simulink model "admire_sim_NDI"  (Simulink 9.1)
settings: Solver=ode4  StartTime=0.0  StopTime=500  FixedStep=dt  RelTol=1e-3  AbsTol=1e-6
InitFcn:
  | INIT_NDI
StartFcn:
  | tic
StopFcn:
  | toctime=toc;
  | fprintf('Actual Time = %g\nSim Time = %g\n',toctime,tout(end))
  | % Make plots
  | %admire_sim_plot
  | figure
  | plot3(yout(:,11),yout(:,10),-yout(:,12),'*-');grid
  | xlabel('East (m)');ylabel('North (m)');zlabel('Alt (m)')
  | view([0 0 1])
  | hold on
  | plot3(Ywpt,Xwpt,0*Xwpt,'r^-','MarkerSize',10)
  | axis equal
  | hold off
values from neighbouring files (symbols this model uses):
  a1 = (180*d2r)/(80^3)    (= 6.13592315154e-06)    [INIT_NDI.m]
  a2 = (24*d2r)/(80^3)    (= 8.18123086872e-07)    [INIT_NDI.m]
  Altcmd_t = [ 0    1   100 200  300  425  450  550  600  700  800  880  980]    [INIT_NDI.m]
  Altcmd_v = [20  20   20   1500 1500 1500 1500 3000 3000 4000 4000 6000 6000]    [INIT_NDI.m]
  bref = 10    [INIT_NDI.m]
  C1 = ((Iy-Iz)*Iz-Ixz^2)/GG    (= -0.958151081688)    [INIT_NDI.m]
  C2 = (Ix-Iy+Iz)*Ixz/GG    (= 0.0484690861804)    [INIT_NDI.m]
  C3 = Iz/GG    (= 4.77597824802e-05)    [INIT_NDI.m]
  C4 = Ixz/GG    (= 1.18217283367e-06)    [INIT_NDI.m]
  C5 = (Iz-Ix)/Iy    (= 0.987654320988)    [INIT_NDI.m]
  C6 = Ixz/Iy    (= 0.0308641975309)    [INIT_NDI.m]
  C7 = 1/Iy    (= 1.23456790123e-05)    [INIT_NDI.m]
  C8 = (Ix*(Ix-Iy)+Ixz^2)/GG    (= -0.592859676085)    [INIT_NDI.m]
  C9 = Ix/GG    (= 9.93025180281e-06)    [INIT_NDI.m]
  CAmethod = 6    [INIT_NDI.m]
  Canard_max = [25 25 25 15 15 15 15 15]*d2r    [INIT_NDI.m]
  Canard_min = [-55 -55 -25 -15 -15 -15 -15 -15]*d2r    [INIT_NDI.m]
  CB = CCV*Bbare    [INIT_NDI.m]
  CC = [C3 0 C4;0 C7 0;C4 0 C9]    [INIT_NDI.m]
  CCV = [CCV zeros(3,22)]    [INIT_NDI.m]
  cref = 5.2    [INIT_NDI.m]
  d2r = pi/180    (= 0.0174532925199)    [INIT_NDI.m]
  dt = 0.01    [INIT_NDI.m]
  DTY_max = 0.002    [INIT_NDI.m]
  DTY_min = -0.002    [INIT_NDI.m]
  DTZ_max = 0.002    [INIT_NDI.m]
  DTZ_min = -0.002    [INIT_NDI.m]
  du = [eye(7,7)*d2r eye(7,7)*(-d2r);zeros(20,14)]    [INIT_NDI.m]
  Elevon_max = [30 30 25 25 25 25 25 25]*d2r    [INIT_NDI.m]
  Elevon_min = [-30 -30 -30 -30 -30 -30 -30 -30]*d2r    [INIT_NDI.m]
  G = [ 0 1 0 ... (first row only)    [INIT_NDI.m]
  kcb = 2.5    [INIT_NDI.m]
  kfb = -0.4    [INIT_NDI.m]
  kib = 0.2    [INIT_NDI.m]
  kpb = 0.8    [INIT_NDI.m]
  LEF_max = [30 30 30 20 20 15 10 10]*d2r    [INIT_NDI.m]
  LEF_min = [-10 -10 -10 -10 -10 -10 -10 -10]*d2r    [INIT_NDI.m]
  LG_max = 1    [INIT_NDI.m]
  LG_min = 0    [INIT_NDI.m]
  LPmethod = 5    [INIT_NDI.m]    (also in LPwrap.m = 0)
  M_vec = [0 0.5 0.8 0.9 0.95 1.4 1.5 2.5]    [INIT_NDI.m]
  mass = 9100    [INIT_NDI.m]
  NumU = 16    [INIT_NDI.m]
  nwpt = 5    [INIT_NDI.m]
  PD_max = 10    [INIT_NDI.m]
  PD_min = -10    [INIT_NDI.m]
  PHIcmd_t = [0 1 1+dt 30 30+dt 60 60+dt 90 90+dt 120 120+dt 150 150+dt 180 180+dt 210 210+dt 240 240+dt 270 270+dt 300 300+dt 330 330+dt]    [INIT_NDI.m]
  PHIcmd_v = [0 0 15   15 -15   -15 0    0   30   30  -30    -30 0      0   45     45   0     0    -45   -45   0     0   -60   -60 0]    [INIT_NDI.m]
  Pmode = 3    [INIT_NDI.m]
  r2d = 180/pi    (= 57.2957795131)    [INIT_NDI.m]
  Rmode = 3    [INIT_NDI.m]
  Rudder_max = [30 30 25 20 15 15 15 10]*d2r    [INIT_NDI.m]
  Rudder_min = [-30 -30 -25 -20 -15 -15 -15 -10]*d2r    [INIT_NDI.m]
  Sref = 45    [INIT_NDI.m]
  TSS_max = 1    [INIT_NDI.m]
  TSS_min = 0    [INIT_NDI.m]
  UD_max = 10    [INIT_NDI.m]
  UD_min = -10    [INIT_NDI.m]
  Upref = [0 0 0 0 0 0 0 0 0 0 0 0 0 0 0 0]'    [INIT_NDI.m]
  Upref_split = [[0 0 30 -30 -30 30 0]*d2r*.4 0 0 0 0 0 0 0 0 0]'    [INIT_NDI.m]
  Urlim = [50*d2r ... (first row only)    [INIT_NDI.m]
  UseRL = 0    [INIT_NDI.m]
  Vcmd_t = [  0    1   100  200  300  425  450  550  600  700  800  880  980]    [INIT_NDI.m]
  Vcmd_v = Mcmd_v.*a    [INIT_NDI.m]
  VD_max = 10    [INIT_NDI.m]
  VD_min = -10    [INIT_NDI.m]
  WD_max = 10    [INIT_NDI.m]
  WD_min = -10    [INIT_NDI.m]
  Wp = W'*W    [INIT_NDI.m]
  Wpts = [0 1 2 3 4]    [INIT_NDI.m]
  x0 = [ max(eyp,zeros(n,1));max(-eyp,zeros(n,1));zeros(2*m,1)]    [LPwrap.m]
  Xwpt = [0 4000 4000 0 0]*8    [INIT_NDI.m]
  Ywpt = [0 0 4000 4000 0]*8    [INIT_NDI.m]
undefined symbols (not defined in the file or in its folder): Abare, Bbare, CGIwrap, dalpha_err, dalt_err, DAwrap, dbeta_err, ddc_bw, ddc_rate, ddei_bw, ddei_rate, ddey_bw, ddey_rate, ddle_bw, ddle_rate, ddr_bw, ddr_rate, DiscIntNeverNeededParam, dVt_err, LPwrap, rlimit_c, rlimit_ie, rlimit_le, rlimit_oe, rlimit_r, u0fcs, u0new, VJAwrap, x0bare, y0bare
libraries: simulink_extras x19, simulink x12
(part 4 of 4)

== system admire_sim_NDI/NDI_CLAW/DynamicInversionControl/AERO_OBM/NonLinearOBM/Get_B_Aero/OneColPerFrame/u4 ==
  In1 : Inport
  Action Port : ActionPort  ActionType=case
  ADMIRE_aerotesthigh : S-Function  FunctionName=admire_aerotesthigh  SFunctionDeploymentMode=off  EnableBusSupport=off
  ADMIRE_aerotesthigh1 : S-Function  FunctionName=admire_aerotesthigh  SFunctionDeploymentMode=off  EnableBusSupport=off
  Constant1 : Constant  Value=zeros(25,1)
  Gain : Gain  Gain=0.5*r2d
  Selector : Selector  NumberOfDimensions=2  InputPortWidth=3  IndexOptions=Index vector (dialog),Index vector (dialog)  Indices=[1:27],4  OutputSizes=1,1
  Selector1 : Selector  NumberOfDimensions=2  InputPortWidth=3  IndexOptions=Index vector (dialog),Index vector (dialog)  Indices=[1:27],11  OutputSizes=1,1
  Selector2 : Selector  InputPortWidth=9  IndexOptions=Index vector (dialog)  Indices=[4:6]  OutputSizes=1
  Selector3 : Selector  InputPortWidth=9  IndexOptions=Index vector (dialog)  Indices=[4:6]  OutputSizes=1
  Sum1 : Sum  Inputs=|+-
  Out1 : Outport
  wires:
  Constant1/1 -> ADMIRE_aerotesthigh/2, ADMIRE_aerotesthigh1/2
  In1/1 -> Selector1/1, Selector/1
  Selector/1 -> ADMIRE_aerotesthigh/1
  Selector1/1 -> ADMIRE_aerotesthigh1/1
  ADMIRE_aerotesthigh/1 -> Selector2/1
  ADMIRE_aerotesthigh1/1 -> Selector3/1
  Sum1/1 -> Gain/1
  Selector2/1 -> Sum1/1
  Selector3/1 -> Sum1/2
  Gain/1 -> Out1/1

== system admire_sim_NDI/NDI_CLAW/DynamicInversionControl/AERO_OBM/NonLinearOBM/Get_B_Aero/OneColPerFrame/u5 ==
  In1 : Inport
  Action Port : ActionPort  ActionType=case
  ADMIRE_aerotesthigh : S-Function  FunctionName=admire_aerotesthigh  SFunctionDeploymentMode=off  EnableBusSupport=off
  ADMIRE_aerotesthigh1 : S-Function  FunctionName=admire_aerotesthigh  SFunctionDeploymentMode=off  EnableBusSupport=off
  Constant1 : Constant  Value=zeros(25,1)
  Gain : Gain  Gain=0.5*r2d
  Selector : Selector  NumberOfDimensions=2  InputPortWidth=3  IndexOptions=Index vector (dialog),Index vector (dialog)  Indices=[1:27],5  OutputSizes=1,1
  Selector1 : Selector  NumberOfDimensions=2  InputPortWidth=3  IndexOptions=Index vector (dialog),Index vector (dialog)  Indices=[1:27],12  OutputSizes=1,1
  Selector2 : Selector  InputPortWidth=9  IndexOptions=Index vector (dialog)  Indices=[4:6]  OutputSizes=1
  Selector3 : Selector  InputPortWidth=9  IndexOptions=Index vector (dialog)  Indices=[4:6]  OutputSizes=1
  Sum1 : Sum  Inputs=|+-
  Out1 : Outport
  wires:
  Gain/1 -> Out1/1
  Selector3/1 -> Sum1/2
  Selector2/1 -> Sum1/1
  Sum1/1 -> Gain/1
  ADMIRE_aerotesthigh1/1 -> Selector3/1
  ADMIRE_aerotesthigh/1 -> Selector2/1
  Selector1/1 -> ADMIRE_aerotesthigh1/1
  Selector/1 -> ADMIRE_aerotesthigh/1
  In1/1 -> Selector/1, Selector1/1
  Constant1/1 -> ADMIRE_aerotesthigh/2, ADMIRE_aerotesthigh1/2

== system admire_sim_NDI/NDI_CLAW/DynamicInversionControl/AERO_OBM/NonLinearOBM/Get_B_Aero/OneColPerFrame/u6 ==
  In1 : Inport
  Action Port : ActionPort  ActionType=case
  ADMIRE_aerotesthigh : S-Function  FunctionName=admire_aerotesthigh  SFunctionDeploymentMode=off  EnableBusSupport=off
  ADMIRE_aerotesthigh1 : S-Function  FunctionName=admire_aerotesthigh  SFunctionDeploymentMode=off  EnableBusSupport=off
  Constant1 : Constant  Value=zeros(25,1)
  Gain : Gain  Gain=0.5*r2d
  Selector : Selector  NumberOfDimensions=2  InputPortWidth=3  IndexOptions=Index vector (dialog),Index vector (dialog)  Indices=[1:27],6  OutputSizes=1,1
  Selector1 : Selector  NumberOfDimensions=2  InputPortWidth=3  IndexOptions=Index vector (dialog),Index vector (dialog)  Indices=[1:27],13  OutputSizes=1,1
  Selector2 : Selector  InputPortWidth=9  IndexOptions=Index vector (dialog)  Indices=[4:6]  OutputSizes=1
  Selector3 : Selector  InputPortWidth=9  IndexOptions=Index vector (dialog)  Indices=[4:6]  OutputSizes=1
  Sum1 : Sum  Inputs=|+-
  Out1 : Outport
  wires:
  Constant1/1 -> ADMIRE_aerotesthigh/2, ADMIRE_aerotesthigh1/2
  In1/1 -> Selector1/1, Selector/1
  Selector/1 -> ADMIRE_aerotesthigh/1
  Selector1/1 -> ADMIRE_aerotesthigh1/1
  ADMIRE_aerotesthigh/1 -> Selector2/1
  ADMIRE_aerotesthigh1/1 -> Selector3/1
  Sum1/1 -> Gain/1
  Selector2/1 -> Sum1/1
  Selector3/1 -> Sum1/2
  Gain/1 -> Out1/1

== system admire_sim_NDI/NDI_CLAW/DynamicInversionControl/AERO_OBM/NonLinearOBM/Get_B_Aero/OneColPerFrame/u7 ==
  In1 : Inport
  Action Port : ActionPort  ActionType=case
  ADMIRE_aerotesthigh : S-Function  FunctionName=admire_aerotesthigh  SFunctionDeploymentMode=off  EnableBusSupport=off
  ADMIRE_aerotesthigh1 : S-Function  FunctionName=admire_aerotesthigh  SFunctionDeploymentMode=off  EnableBusSupport=off
  Constant1 : Constant  Value=zeros(25,1)
  Gain : Gain  Gain=0.5*r2d
  Selector : Selector  NumberOfDimensions=2  InputPortWidth=3  IndexOptions=Index vector (dialog),Index vector (dialog)  Indices=[1:27],7  OutputSizes=1,1
  Selector1 : Selector  NumberOfDimensions=2  InputPortWidth=3  IndexOptions=Index vector (dialog),Index vector (dialog)  Indices=[1:27],14  OutputSizes=1,1
  Selector2 : Selector  InputPortWidth=9  IndexOptions=Index vector (dialog)  Indices=[4:6]  OutputSizes=1
  Selector3 : Selector  InputPortWidth=9  IndexOptions=Index vector (dialog)  Indices=[4:6]  OutputSizes=1
  Sum1 : Sum  Inputs=|+-
  Out1 : Outport
  wires:
  Gain/1 -> Out1/1
  Selector3/1 -> Sum1/2
  Selector2/1 -> Sum1/1
  Sum1/1 -> Gain/1
  ADMIRE_aerotesthigh1/1 -> Selector3/1
  ADMIRE_aerotesthigh/1 -> Selector2/1
  Selector1/1 -> ADMIRE_aerotesthigh1/1
  Selector/1 -> ADMIRE_aerotesthigh/1
  In1/1 -> Selector/1, Selector1/1
  Constant1/1 -> ADMIRE_aerotesthigh/2, ADMIRE_aerotesthigh1/2

== system admire_sim_NDI/NDI_CLAW/DynamicInversionControl/ControlAllocation/GetU/WeightedPseudo Scaled_2/Blocks/CheckSaturation ==
  In1 : Inport
  Umin : Inport  Port=2
  Umax : Inport  Port=3
  Relational Operator : RelationalOperator  Operator=<  OutDataTypeStr=boolean  RndMeth=Nearest
  Relational Operator1 : RelationalOperator  Operator=>  OutDataTypeStr=boolean  RndMeth=Nearest
  Sum : Sum  Inputs=|++
  Sum of Elements : Sum  Inputs=+
  Sum of Elements1 : Sum  Inputs=+
  Out1 : Outport
  wires:
  Sum/1 -> Out1/1
  In1/1 -> Relational Operator/1, Relational Operator1/1
  Sum of Elements1/1 -> Sum/2
  Sum of Elements/1 -> Sum/1
  Relational Operator/1 -> Sum of Elements1/1
  Relational Operator1/1 -> Sum of Elements/1
  Umax/1 -> Relational Operator1/2
  Umin/1 -> Relational Operator/2

== system admire_sim_NDI/NDI_CLAW/DynamicInversionControl/ControlAllocation/GetU/WeightedPseudo Scaled_2/Blocks/GetP ==
  CB : Inport
  WpT : Inport  Port=2
  CBT : Inport  Port=3
  Product : Product  Inputs=/*  Multiplication=Matrix(*)  RndMeth=Zero
  Product1 : Product  Inputs=**  Multiplication=Matrix(*)  RndMeth=Zero
  Product2 : Product  Inputs=*/  Multiplication=Matrix(*)  RndMeth=Zero
  P : Outport
  wires:
  CBT/1 -> Product/2
  Product2/1 -> P/1  "P"
  WpT/1 -> Product/1
  CB/1 -> Product1/1
  Product1/1 -> Product2/2
  Product/1 -> Product2/1, Product1/2

== system admire_sim_NDI/NDI_CLAW/DynamicInversionControl/ControlAllocation/GetU/WeightedPseudo Scaled_2/Blocks/None_Saturated ==
  In1 : Inport
  Action Port : ActionPort  ActionType=then
  Out1 : Outport
  wires:
  In1/1 -> Out1/1

== system admire_sim_NDI/NDI_CLAW/DynamicInversionControl/ControlAllocation/GetU/WeightedPseudo Scaled_2/Blocks/Some_Saturated ==
  umax : Inport
  umin : Inport  Port=2
  u : Inport  Port=3
  Action Port : ActionPort  ActionType=else
  For Iterator Subsystem : Subsystem  TreatAsAtomicUnit=on
  Product : Product  RndMeth=Zero
  Out1 : Outport
  wires:
  Product/1 -> Out1/1
  For Iterator Subsystem/1(Out1) -> Product/2
  umin/1 -> For Iterator Subsystem/3(umin)
  umax/1 -> For Iterator Subsystem/2(umax)
  u/1 -> Product/1, For Iterator Subsystem/1(u)

== system admire_sim_NDI/NDI_CLAW/DynamicInversionControl/ControlAllocation/PostProcess/DriveToPreferred/LimitScale/Calculate the gain factor to the lower limit  ==
  oou : Inport
  MaxValues : Inport  Port=2
  PrePro : Inport  Port=3
  Bus Selector2 : BusSelector  OutputSignals=INDX
  Compare To Constant : simulink/Logic and Bit Operations/Compare To Constant  relop=<=  const=0.5  OutDataTypeStr=uint8
  Data Type Conversion : DataTypeConversion  OutDataTypeStr=double
  Product : Product  Inputs=*/  RndMeth=Zero
  Product2 : Product
  Sum : Sum  Inputs=|++
  Out1 : Outport
  wires:
  Compare To Constant/1 -> Data Type Conversion/1
  Data Type Conversion/1 -> Sum/1
  Bus Selector2/1 -> Product2/1, Compare To Constant/1  "<INDX>"
  Product2/1 -> Sum/2
  PrePro/1 -> Bus Selector2/1
  MaxValues/1 -> Product/1
  Sum/1 -> Out1/1
  oou/1 -> Product/2
  Product/1 -> Product2/2  "gain,  K"

== system admire_sim_NDI/NDI_CLAW/DynamicInversionControl/ControlAllocation/PostProcess/DriveToPreferred/LimitScale/Calculate the gain factor to the upper limit  ==
  PrePro : Inport
  MinValues : Inport  Port=2
  oou : Inport  Port=3
  Bus Selector2 : BusSelector  OutputSignals=INDX
  Compare To Constant : simulink/Logic and Bit Operations/Compare To Constant  relop=<=  const=0.5  OutDataTypeStr=uint8
  Data Type Conversion : DataTypeConversion  OutDataTypeStr=double
  Product : Product  Inputs=*/  RndMeth=Zero
  Product2 : Product
  Sum : Sum  Inputs=|++
  Out1 : Outport
  wires:
  Product/1 -> Product2/2
  oou/1 -> Product/2
  Sum/1 -> Out1/1
  MinValues/1 -> Product/1
  PrePro/1 -> Bus Selector2/1
  Product2/1 -> Sum/2
  Bus Selector2/1 -> Product2/1, Compare To Constant/1  "<INDX>"
  Data Type Conversion/1 -> Sum/1
  Compare To Constant/1 -> Data Type Conversion/1

== system admire_sim_NDI/NDI_CLAW/DynamicInversionControl/ControlAllocation/PostProcess/DriveToPreferred/LimitScale/DivideByZeroProtection ==
  In1 : Inport
  Abs : Abs
  Compare To Constant : simulink/Logic and Bit Operations/Compare To Constant  relop=<=  const=1e-5  OutDataTypeStr=uint8
  Compare To Zero : simulink/Logic and Bit Operations/Compare To Zero  relop=>=  OutDataTypeStr=uint8
  Constant : Constant
  Data Type Conversion : DataTypeConversion  OutDataTypeStr=double
  Data Type Conversion1 : DataTypeConversion  OutDataTypeStr=double
  Gain1 : Gain  Gain=1e-5
  Gain2 : Gain  Gain=2
  Product1 : Product  RndMeth=Zero
  Sum : Sum  Inputs=|++
  Sum1 : Sum  Inputs=|+-
  Out1 : Outport
  wires:
  Abs/1 -> Compare To Constant/1
  Data Type Conversion/1 -> Gain1/1
  Gain1/1 -> Product1/1
  Sum1/1 -> Data Type Conversion1/1
  Compare To Zero/1 -> Gain2/1
  Gain2/1 -> Sum1/1
  Constant/1 -> Sum1/2
  Data Type Conversion1/1 -> Product1/2
  Compare To Constant/1 -> Data Type Conversion/1
  In1/1 -> Sum/1, Compare To Zero/1, Abs/1
  Product1/1 -> Sum/2
  Sum/1 -> Out1/1

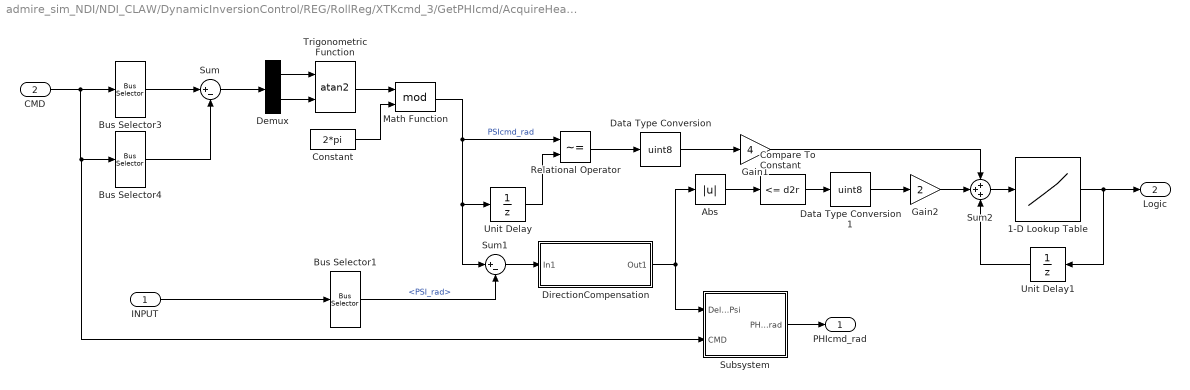
== system admire_sim_NDI/NDI_CLAW/DynamicInversionControl/REG/RollReg/XTKcmd_3/GetPHIcmd/AcquireHeading ==
  INPUT : Inport
  CMD : Inport  Port=2
  1-D Lookup Table : Lookup_n-D  NumberOfTableDimensions=1  BreakpointsForDimension1=[0 1 2 3 4 5 6 7]  Table=[0 1 0 0 1 1 1 1]  InterpMethod=Flat  OutDataTypeStr=uint8  RndMeth=Simplest  InputSameDT=on
  Abs : Abs
  Bus Selector1 : BusSelector  OutputSignals=PSI_rad
  Bus Selector3 : BusSelector  OutputSignals=Ycmd,Xcmd  OutputAsBus=on
  Bus Selector4 : BusSelector  OutputSignals=Ycmdm1,Xcmdm1  OutputAsBus=on
  Compare To Constant : simulink/Logic and Bit Operations/Compare To Constant  relop=<=  const=d2r  OutDataTypeStr=uint8
  Constant : Constant  Value=2*pi
  Data Type Conversion : DataTypeConversion  OutDataTypeStr=uint8
  Data Type Conversion1 : DataTypeConversion  OutDataTypeStr=uint8
  Demux : Demux  Outputs=2
  DirectionCompensation : Subsystem
  Gain1 : Gain  Gain=4  OutDataTypeStr=uint8
  Gain2 : Gain  Gain=2  OutDataTypeStr=uint8
  Math Function : Math  Operator=mod  SaturateOnIntegerOverflow=on
  Relational Operator : RelationalOperator  Operator=~=  OutDataTypeStr=boolean  RndMeth=Nearest
  Subsystem : Subsystem
  Sum : Sum  Inputs=|+-
  Sum1 : Sum  Inputs=|+-
  Sum2 : Sum  Inputs=+++
  Trigonometric Function : Trigonometry  Operator=atan2
  Unit Delay : UnitDelay  SampleTime=-1
  Unit Delay1 : UnitDelay  SampleTime=-1
  PHIcmd_rad : Outport
  Logic : Outport  Port=2
  wires:
  CMD/1 -> Subsystem/2(CMD), Bus Selector4/1, Bus Selector3/1
  INPUT/1 -> Bus Selector1/1
  Bus Selector3/1 -> Sum/1
  Bus Selector4/1 -> Sum/2
  Sum/1 -> Demux/1
  Demux/1 -> Trigonometric Function/1
  Demux/2 -> Trigonometric Function/2
  Trigonometric Function/1 -> Math Function/1
  Bus Selector1/1 -> Sum1/2  "<PSI_rad>"
  Math Function/1 -> Unit Delay/1, Sum1/1, Relational Operator/1  "PSIcmd_rad"
  Sum1/1 -> DirectionCompensation/1(In1)
  DirectionCompensation/1(Out1) -> Subsystem/1(DeltaPsi), Abs/1
  Constant/1 -> Math Function/2
  Unit Delay/1 -> Relational Operator/2
  Relational Operator/1 -> Data Type Conversion/1
  Abs/1 -> Compare To Constant/1
  Compare To Constant/1 -> Data Type Conversion1/1
  Sum2/1 -> 1-D Lookup Table/1
  Data Type Conversion/1 -> Gain1/1
  Gain1/1 -> Sum2/1
  Gain2/1 -> Sum2/2
  Data Type Conversion1/1 -> Gain2/1
  Unit Delay1/1 -> Sum2/3
  1-D Lookup Table/1 -> Logic/1, Unit Delay1/1
  Subsystem/1(PHIcmd_rad) -> PHIcmd_rad/1

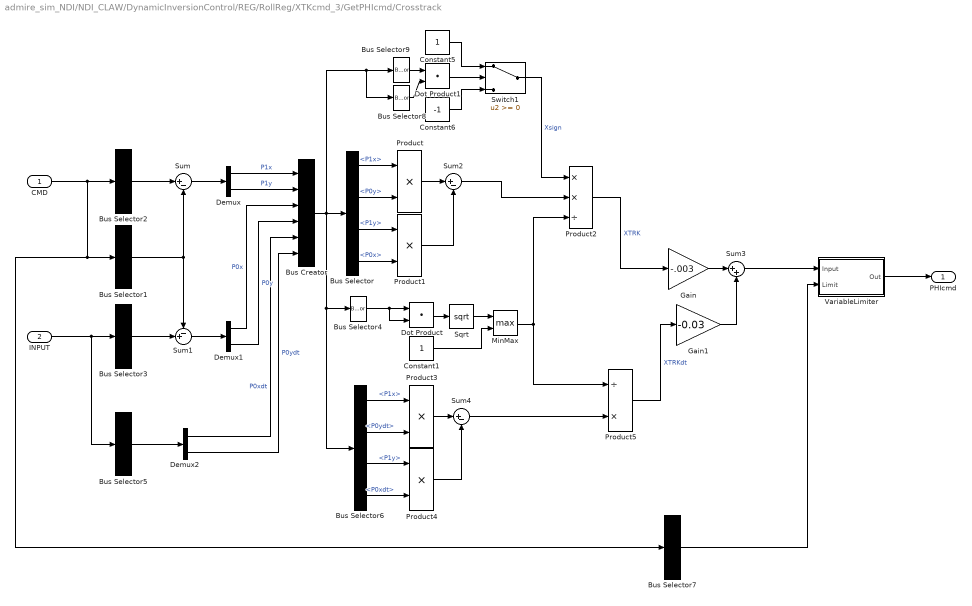
== system admire_sim_NDI/NDI_CLAW/DynamicInversionControl/REG/RollReg/XTKcmd_3/GetPHIcmd/Crosstrack ==
  CMD : Inport
  INPUT : Inport  Port=2
  Bus Creator : BusCreator  Inputs=6
  Bus Selector : BusSelector  OutputSignals=P1x,P0y,P1y,P0x
  Bus Selector1 : BusSelector  OutputSignals=Xcmdm1,Ycmdm1  OutputAsBus=on
  Bus Selector2 : BusSelector  OutputSignals=Xcmd,Ycmd  OutputAsBus=on
  Bus Selector3 : BusSelector  OutputSignals=X_m,Y_m  OutputAsBus=on
  Bus Selector4 : BusSelector  OutputSignals=P1x,P1y  OutputAsBus=on
  Bus Selector5 : BusSelector  OutputSignals=XV_mps,YV_mps  OutputAsBus=on
  Bus Selector6 : BusSelector  OutputSignals=P1x,P0ydt,P1y,P0xdt
  Bus Selector7 : BusSelector  OutputSignals=PHImax_rad  OutputAsBus=on
  Bus Selector8 : BusSelector  OutputSignals=P0xdt,P0ydt  OutputAsBus=on
  Bus Selector9 : BusSelector  OutputSignals=P1x,P1y  OutputAsBus=on
  Constant1 : Constant
  Constant5 : Constant
  Constant6 : Constant  Value=-1
  Demux : Demux  Outputs=2
  Demux1 : Demux  Outputs=2
  Demux2 : Demux  Outputs=2
  Dot Product : DotProduct  InputSameDT=on  OutDataTypeStr=Inherit: Inherit via internal rule
  Dot Product1 : DotProduct  InputSameDT=on  OutDataTypeStr=Inherit: Inherit via internal rule
  Gain : Gain  Gain=-.003
  Gain1 : Gain  Gain=-0.03
  MinMax : MinMax  Function=max  Inputs=2
  Product{,1,3..4} (4 alike) : Product  RndMeth=Zero
  Product2 : Product  Inputs=**/  RndMeth=Zero
  Product5 : Product  Inputs=/*  RndMeth=Zero
  Sqrt : Sqrt  SaturateOnIntegerOverflow=on
  Sum : Sum  Inputs=|+-
  Sum1 : Sum  Inputs=-+|
  Sum2 : Sum  Inputs=|+-
  Sum3 : Sum  Inputs=|++
  Sum4 : Sum  Inputs=|+-
  Switch1 : Switch
  VariableLimiter : Subsystem
  PHIcmd : Outport
  wires:
  CMD/1 -> Bus Selector2/1, Bus Selector1/1, Bus Selector7/1
  Bus Selector2/1 -> Sum/1
  Bus Selector1/1 -> Sum/2, Sum1/1
  INPUT/1 -> Bus Selector3/1, Bus Selector5/1
  Bus Selector3/1 -> Sum1/2
  Sum/1 -> Demux/1
  Sum1/1 -> Demux1/1
  Demux/1 -> Bus Creator/1  "P1x"
  Demux/2 -> Bus Creator/2  "P1y"
  Demux1/1 -> Bus Creator/3  "P0x"
  Demux1/2 -> Bus Creator/4  "P0y"
  Bus Creator/1 -> Bus Selector/1, Bus Selector4/1, Bus Selector6/1, Bus Selector9/1, Bus Selector8/1
  Bus Selector/1 -> Product/1  "<P1x>"
  Bus Selector/2 -> Product/2  "<P0y>"
  Bus Selector/3 -> Product1/1  "<P1y>"
  Bus Selector/4 -> Product1/2  "<P0x>"
  Product/1 -> Sum2/1
  Product1/1 -> Sum2/2
  Bus Selector4/1 -> Dot Product/1, Dot Product/2
  Dot Product/1 -> Sqrt/1
  Sqrt/1 -> MinMax/1
  Constant1/1 -> MinMax/2
  MinMax/1 -> Product5/1, Product2/3
  Product2/1 -> Gain/1  "XTRK"
  Gain/1 -> Sum3/1
  Bus Selector5/1 -> Demux2/1
  Demux2/1 -> Bus Creator/5  "P0xdt"
  Demux2/2 -> Bus Creator/6  "P0ydt"
  Bus Selector6/1 -> Product3/1  "<P1x>"
  Bus Selector6/2 -> Product3/2  "<P0ydt>"
  Bus Selector6/3 -> Product4/1  "<P1y>"
  Bus Selector6/4 -> Product4/2  "<P0xdt>"
  Product3/1 -> Sum4/1
  Product4/1 -> Sum4/2
  Sum4/1 -> Product5/2
  Gain1/1 -> Sum3/2
  Sum3/1 -> VariableLimiter/1(Input)
  VariableLimiter/1(Out) -> PHIcmd/1
  Product5/1 -> Gain1/1  "XTRKdt"
  Sum2/1 -> Product2/2
  Constant5/1 -> Switch1/1
  Constant6/1 -> Switch1/3
  Bus Selector9/1 -> Dot Product1/1
  Bus Selector8/1 -> Dot Product1/2
  Dot Product1/1 -> Switch1/2
  Bus Selector7/1 -> VariableLimiter/2(Limit)
  Switch1/1 -> Product2/1  "Xsign"

== system admire_sim_NDI/NDI_CLAW/DynamicInversionControl/AERO_OBM/NonLinearOBM/Get_B_Aero/Get_CVdt/TotalAccels/Get_Pbdt1 ==
  In1 : Inport
  Bus Selector : BusSelector  OutputSignals=Rb,Pb,Qb,Mx,Mz
  Gain : Gain  Gain=C1
  Gain1 : Gain  Gain=C2
  Gain2 : Gain  Gain=C3
  Gain3 : Gain  Gain=C4
  Product : Product  RndMeth=Zero
  Sum : Sum  Inputs=|++
  Sum1 : Sum  Inputs=+++
  Pbdt : Outport
  wires:
  Sum1/1 -> Pbdt/1  "Pbdt_rps2"
  In1/1 -> Bus Selector/1
  Gain3/1 -> Sum1/3
  Product/1 -> Sum1/1
  Gain2/1 -> Sum1/2
  Bus Selector/5 -> Gain3/1  "<Mz>"
  Bus Selector/4 -> Gain2/1  "<Mx>"
  Bus Selector/3 -> Product/2  "<Qb>"
  Sum/1 -> Product/1
  Gain1/1 -> Sum/2
  Gain/1 -> Sum/1
  Bus Selector/2 -> Gain1/1  "<Pb>"
  Bus Selector/1 -> Gain/1  "<Rb>"

== system admire_sim_NDI/NDI_CLAW/DynamicInversionControl/AERO_OBM/NonLinearOBM/Get_B_Aero/Get_CVdt/TotalAccels/Get_Qbdt1 ==
  In1 : Inport
  Bus Selector : BusSelector  OutputSignals=Pb,Rb,Pb,Rb,My
  Gain4 : Gain  Gain=C5
  Gain5 : Gain  Gain=C6
  Gain6 : Gain  Gain=C7
  Product1 : Product  RndMeth=Zero
  Product2 : Product  RndMeth=Zero
  Product3 : Product  RndMeth=Zero
  Sum1 : Sum  Inputs=+-+
  Sum2 : Sum  Inputs=|+-
  Qbdt : Outport
  wires:
  Gain6/1 -> Sum1/3
  Gain5/1 -> Sum1/2
  Gain4/1 -> Sum1/1
  Bus Selector/5 -> Gain6/1  "<My>"
  Sum2/1 -> Gain5/1
  Product3/1 -> Sum2/2
  Product2/1 -> Sum2/1
  Bus Selector/4 -> Product3/2, Product3/1  "<Rb>"
  Bus Selector/3 -> Product2/2, Product2/1  "<Pb>"
  Product1/1 -> Gain4/1
  Bus Selector/2 -> Product1/2  "<Rb>"
  Bus Selector/1 -> Product1/1  "<Pb>"
  In1/1 -> Bus Selector/1
  Sum1/1 -> Qbdt/1  "Qbdt_rps2"

== system admire_sim_NDI/NDI_CLAW/DynamicInversionControl/AERO_OBM/NonLinearOBM/Get_B_Aero/Get_CVdt/TotalAccels/Get_Rbdt1 ==
  In1 : Inport
  Bus Selector : BusSelector  OutputSignals=Pb,Rb,Qb,Mx,Mz
  Gain : Gain  Gain=C8
  Gain1 : Gain  Gain=C2
  Gain2 : Gain  Gain=C4
  Gain3 : Gain  Gain=C9
  Product : Product  RndMeth=Zero
  Sum : Sum  Inputs=|+-
  Sum1 : Sum  Inputs=+++
  Rbdt : Outport
  wires:
  Bus Selector/5 -> Gain3/1  "<Mz>"
  Bus Selector/4 -> Gain2/1  "<Mx>"
  Bus Selector/3 -> Product/2  "<Qb>"
  Bus Selector/2 -> Gain1/1  "<Rb>"
  Bus Selector/1 -> Gain/1  "<Pb>"
  Sum1/1 -> Rbdt/1  "Rbdt_rps2"
  In1/1 -> Bus Selector/1
  Gain3/1 -> Sum1/3
  Product/1 -> Sum1/1
  Gain2/1 -> Sum1/2
  Sum/1 -> Product/1
  Gain1/1 -> Sum/2
  Gain/1 -> Sum/1

== system admire_sim_NDI/NDI_CLAW/DynamicInversionControl/ControlAllocation/GetU/WeightedPseudo Scaled_2/Blocks/Some_Saturated/For Iterator Subsystem ==
  u : Inport
  umax : Inport  Port=2
  umin : Inport  Port=3
  Bus Creator : BusCreator  Inputs=3
  Bus Selector : BusSelector  OutputSignals=uidx,umaxidx,uminidx
  Bus Selector1 : BusSelector  OutputSignals=uidx,umaxidx
  Bus Selector2 : BusSelector  OutputSignals=uidx,uminidx
  For Iterator : ForIterator  IterationLimit=7
  Gain : Gain
  If : If  NumInputs=3  IfExpression=u1 > u2  ElseIfExpressions=u1 < u3
  If Action Subsystem : Subsystem  TreatAsAtomicUnit=on
  If Action Subsystem1 : Subsystem  TreatAsAtomicUnit=on
  If Action Subsystem2 : Subsystem  TreatAsAtomicUnit=on
  Merge : Merge  Inputs=3
  Selector : Selector  IndexOptions=Index vector (port)  Indices=[1 3]  OutputSizes=1
  Selector1 : Selector  IndexOptions=Index vector (port)  Indices=[1 3]  OutputSizes=1
  Selector2 : Selector  IndexOptions=Index vector (port)  Indices=[1 3]  OutputSizes=1
  Unit Delay : UnitDelay  InitialCondition=1  SampleTime=-1
  Out1 : Outport
  wires:
  Bus Selector2/2 -> If Action Subsystem1/2(ulim)  "<uminidx>"
  Bus Selector2/1 -> If Action Subsystem1/1(u)  "<uidx>"
  Bus Selector1/2 -> If Action Subsystem2/2(ulim)  "<umaxidx>"
  Bus Selector1/1 -> If Action Subsystem2/1(u)  "<uidx>"
  Bus Selector/3 -> If/3  "<uminidx>"
  Bus Selector/2 -> If/2  "<umaxidx>"
  Bus Selector/1 -> If/1  "<uidx>"
  Bus Creator/1 -> Bus Selector2/1, Bus Selector1/1, Bus Selector/1
  Unit Delay/1 -> If Action Subsystem1/3(scale_z), If Action Subsystem/1(In1), If Action Subsystem2/3(scale_z)
  Merge/1 -> Unit Delay/1, Gain/1
  If Action Subsystem1/1(Out1) -> Merge/2
  If Action Subsystem2/1(Out1) -> Merge/3
  If Action Subsystem/1(Out1) -> Merge/1
  If/1 -> If Action Subsystem2/Action
  If/2 -> If Action Subsystem1/Action
  If/3 -> If Action Subsystem/Action
  Selector2/1 -> Bus Creator/3  "uminidx"
  Selector1/1 -> Bus Creator/2  "umaxidx"
  Selector/1 -> Bus Creator/1  "uidx"
  umin/1 -> Selector2/1
  umax/1 -> Selector1/1
  Gain/1 -> Out1/1
  For Iterator/1 -> Selector2/2, Selector1/2, Selector/2
  u/1 -> Selector/1

== system admire_sim_NDI/NDI_CLAW/DynamicInversionControl/REG/RollReg/XTKcmd_3/GetPHIcmd/AcquireHeading/DirectionCompensation ==
  In1 : Inport
  Compare To Constant : simulink/Logic and Bit Operations/Compare To Constant  relop=<=  const=pi  OutDataTypeStr=uint8
  Compare To Constant1 : simulink/Logic and Bit Operations/Compare To Constant  relop=>=  const=-pi  OutDataTypeStr=uint8
  Constant1 : Constant  Value=2*pi
  Constant2 : Constant  Value=2*pi
  Sum : Sum  Inputs=|+-
  Sum1 : Sum  Inputs=|++
  Switch : Switch  Criteria=u2 > Threshold
  Switch1 : Switch
  Switch2 : Switch  Criteria=u2 > Threshold
  Out1 : Outport
  wires:
  Constant2/1 -> Sum1/2
  Sum1/1 -> Switch2/3
  Switch2/1 -> Switch1/3
  Compare To Constant1/1 -> Switch2/2
  Switch/1 -> Switch1/1
  Sum/1 -> Switch/3
  Constant1/1 -> Sum/2
  Compare To Constant/1 -> Switch/2
  In1/1 -> Switch1/2, Switch2/1, Sum1/1, Compare To Constant1/1, Sum/1, Compare To Constant/1, Switch/1
  Switch1/1 -> Out1/1

== system admire_sim_NDI/NDI_CLAW/DynamicInversionControl/REG/RollReg/XTKcmd_3/GetPHIcmd/AcquireHeading/Subsystem ==
  DeltaPsi : Inport
  CMD : Inport  Port=2
  Bus Selector2 : BusSelector  OutputSignals=PHImax_rad
  Gain6 : Gain  Gain=-1
  Switch1 : Switch
  PHIcmd_rad : Outport
  wires:
  Gain6/1 -> Switch1/3
  Bus Selector2/1 -> Gain6/1, Switch1/1  "<PHImax_rad>"
  Switch1/1 -> PHIcmd_rad/1
  CMD/1 -> Bus Selector2/1
  DeltaPsi/1 -> Switch1/2

== system admire_sim_NDI/NDI_CLAW/DynamicInversionControl/REG/RollReg/XTKcmd_3/GetPHIcmd/Crosstrack/VariableLimiter ==
  Input : Inport
  Limit : Inport  Port=2
  Gain : Gain  Gain=-1
  MinMax : MinMax  Inputs=2
  MinMax1 : MinMax  Function=max  Inputs=2
  Out : Outport
  wires:
  MinMax1/1 -> Out/1
  Limit/1 -> Gain/1, MinMax/2
  Input/1 -> MinMax/1
  Gain/1 -> MinMax1/2
  MinMax/1 -> MinMax1/1

== system admire_sim_NDI/NDI_CLAW/DynamicInversionControl/ControlAllocation/GetU/WeightedPseudo Scaled_2/Blocks/Some_Saturated/For Iterator Subsystem/If Action Subsystem ==
  In1 : Inport
  Action Port : ActionPort  ActionType=else
  Out1 : Outport
  wires:
  In1/1 -> Out1/1

== system admire_sim_NDI/NDI_CLAW/DynamicInversionControl/ControlAllocation/GetU/WeightedPseudo Scaled_2/Blocks/Some_Saturated/For Iterator Subsystem/If Action Subsystem1 ==
  u : Inport
  ulim : Inport  Port=2
  scale_z : Inport  Port=3
  Action Port : ActionPort  ActionType=elseif
  Abs : Abs
  If : If  IfExpression=u1 >1e-5
  If Action Subsystem : Subsystem  TreatAsAtomicUnit=on
  If Action Subsystem1 : Subsystem  TreatAsAtomicUnit=on
  Merge : Merge
  Out1 : Outport
  wires:
  If Action Subsystem/1(Out1) -> Merge/2
  If/1 -> If Action Subsystem/Action
  If Action Subsystem1/1(Out1) -> Merge/1
  If/2 -> If Action Subsystem1/Action
  scale_z/1 -> If Action Subsystem/3(scale_z)
  ulim/1 -> If Action Subsystem/2(ulim)
  Merge/1 -> Out1/1
  u/1 -> If Action Subsystem/1(u), Abs/1
  Abs/1 -> If/1

== system admire_sim_NDI/NDI_CLAW/DynamicInversionControl/ControlAllocation/GetU/WeightedPseudo Scaled_2/Blocks/Some_Saturated/For Iterator Subsystem/If Action Subsystem2 ==
  u : Inport
  ulim : Inport  Port=2
  scale_z : Inport  Port=3
  Action Port : ActionPort  ActionType=then
  Abs : Abs
  If : If  IfExpression=u1 >1e-5
  If Action Subsystem : Subsystem  TreatAsAtomicUnit=on
  If Action Subsystem1 : Subsystem  TreatAsAtomicUnit=on
  Merge : Merge
  Out1 : Outport
  wires:
  If Action Subsystem/1(Out1) -> Merge/2
  If/1 -> If Action Subsystem/Action
  If Action Subsystem1/1(Out1) -> Merge/1
  If/2 -> If Action Subsystem1/Action
  scale_z/1 -> If Action Subsystem/3(scale_z)
  ulim/1 -> If Action Subsystem/2(ulim)
  Merge/1 -> Out1/1
  u/1 -> If Action Subsystem/1(u), Abs/1
  Abs/1 -> If/1

== system admire_sim_NDI/NDI_CLAW/DynamicInversionControl/ControlAllocation/GetU/WeightedPseudo Scaled_2/Blocks/Some_Saturated/For Iterator Subsystem/If Action Subsystem1/If Action Subsystem ==
  u : Inport
  ulim : Inport  Port=2
  scale_z : Inport  Port=3
  Action Port : ActionPort  ActionType=then
  MinMax : MinMax  Inputs=2
  Product : Product  Inputs=*/  RndMeth=Zero
  Out1 : Outport
  wires:
  MinMax/1 -> Out1/1
  Product/1 -> MinMax/1
  u/1 -> Product/2
  ulim/1 -> Product/1
  scale_z/1 -> MinMax/2

== system admire_sim_NDI/NDI_CLAW/DynamicInversionControl/ControlAllocation/GetU/WeightedPseudo Scaled_2/Blocks/Some_Saturated/For Iterator Subsystem/If Action Subsystem1/If Action Subsystem1 ==
  Action Port : ActionPort  ActionType=else
  Constant4 : Constant  Value=0
  Out1 : Outport
  wires:
  Constant4/1 -> Out1/1

== system admire_sim_NDI/NDI_CLAW/DynamicInversionControl/ControlAllocation/GetU/WeightedPseudo Scaled_2/Blocks/Some_Saturated/For Iterator Subsystem/If Action Subsystem2/If Action Subsystem ==
  u : Inport
  ulim : Inport  Port=2
  scale_z : Inport  Port=3
  Action Port : ActionPort  ActionType=then
  MinMax : MinMax  Inputs=2
  Product : Product  Inputs=*/  RndMeth=Zero
  Out1 : Outport
  wires:
  MinMax/1 -> Out1/1
  Product/1 -> MinMax/1
  u/1 -> Product/2
  ulim/1 -> Product/1
  scale_z/1 -> MinMax/2

== system admire_sim_NDI/NDI_CLAW/DynamicInversionControl/ControlAllocation/GetU/WeightedPseudo Scaled_2/Blocks/Some_Saturated/For Iterator Subsystem/If Action Subsystem2/If Action Subsystem1 ==
  Action Port : ActionPort  ActionType=else
  Constant4 : Constant  Value=0
  Out1 : Outport
  wires:
  Constant4/1 -> Out1/1
